simulink model "sistim"  (R2016a)
settings: Solver=FixedStepAuto  StartTime=0.0  StopTime=10.0  RelTol=1e-3
undefined symbols (not defined in the file): intellegent_control, LED_control, sigbuilder_block
libraries: fuzblock x2
settings Model: Creator=USER  LastModifiedBy=USER

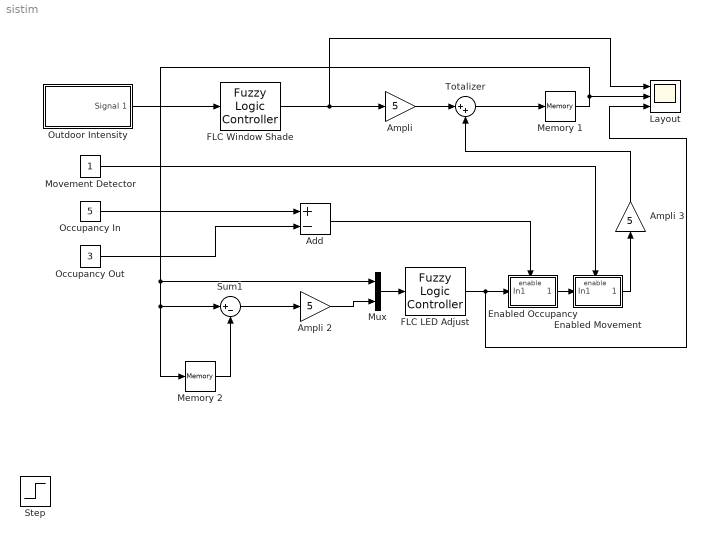
== system sistim ==
  "                     Totalizer" : Sum  Inputs=|++
  Add : Sum  Inputs=+-
  Ampli : Gain  Gain=5
  Ampli 2 : Gain  Gain=5
  Ampli 3 : Gain  Gain=5
  Enabled Movement : Subsystem  TreatAsAtomicUnit=on
  Enabled Occupancy : Subsystem  TreatAsAtomicUnit=on
  FLC LED Adjust : fuzblock/Fuzzy Logic  Controller  fis=[LED_control]
  FLC Window Shade : fuzblock/Fuzzy Logic  Controller  fis=[intellegent_control]
  Layout : Scope  NumInputPorts=3
  Memory 1 : Memory
  Memory 2 : Memory
  "Movement Detector " : Constant
  Mux : Mux  Inputs=2
  "Occupancy In " : Constant  Value=5
  Occupancy Out : Constant  Value=3
  Outdoor Intensity : Subsystem  Tag=STV Subsys  LoadFcn=sigbuilder_block('load');  StartFcn=sigbuilder_block('start');  StopFcn=sigbuilder_block('stop');  ClipboardFcn=sigbuilder_block('clipboard');  mask(Sigbuilder block){}
      mask help: Simulink:masks:SigbuilderBlock_MD
      mask init:
      | if ~strcmp(get_param(bdroot(gcbh),'SimulationStatus'),'stopped') tuvar = sigbuilder_block('maskInit'); end
      settings: CopyFcn=sigbuilder_block('copy');  DeleteFcn=sigbuilder_block('delete');  ModelCloseFcn=sigbuilder_block('modelClose');  PreSaveFcn=sigbuilder_block('preSave');  PauseFcn=sigbuilder_block('pause');  ContinueFcn=sigbuilder_block('continue');  NameChangeFcn=sigbuilder_block('namechange');  OpenFcn=sigbuilder_block('open',[317.25 117 550.5 359.25 ]);  CloseFcn=sigbuilder_block('close');
      mask Display: plot(0, 0, 100, 100,[2, 2, 32, 32, 2], [68, 8, 8, 68, 68],[32, 2], [38, 38], [32, 19, 2],[53, 60, 44], [32, 17, 17, 2],[16, 16, 31, 31]);txt = getActiveGroup(gcbh);text(2, 100, txt,'verticalAlignment', 'top');
  Step : Step  SampleTime=0
  Sum1 : Sum  Inputs=|+-
  wires:
  FLC Window Shade/1 -> Layout/1, Ampli/1
  "                     Totalizer"/1 -> Memory 1/1
  "Occupancy In "/1 -> Add/1
  Occupancy Out/1 -> Add/2
  Enabled Occupancy/1(Out1) -> Enabled Movement/1(In1)
  Add/1 -> Enabled Occupancy/Enable
  "Movement Detector "/1 -> Enabled Movement/Enable
  Mux/1 -> FLC LED Adjust/1
  Memory 2/1 -> Sum1/2
  Memory 1/1 -> Layout/2, Memory 2/1, Sum1/1, Mux/1
  Ampli 2/1 -> Mux/2
  Sum1/1 -> Ampli 2/1
  Enabled Movement/1(Out1) -> Ampli 3/1
  Ampli 3/1 -> "                     Totalizer"/2
  Ampli/1 -> "                     Totalizer"/1
  FLC LED Adjust/1 -> Layout/3, Enabled Occupancy/1(In1)
  Outdoor Intensity/1(Signal 1) -> FLC Window Shade/1

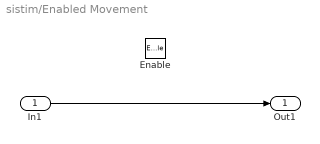
== system sistim/Enabled Movement ==
  In1 : Inport
  Enable : EnablePort
  Out1 : Outport
  wires:
  In1/1 -> Out1/1

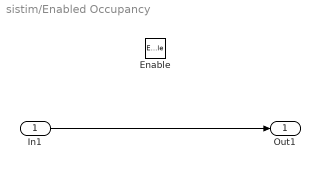
== system sistim/Enabled Occupancy ==
  In1 : Inport
  Enable : EnablePort
  Out1 : Outport
  wires:
  In1/1 -> Out1/1

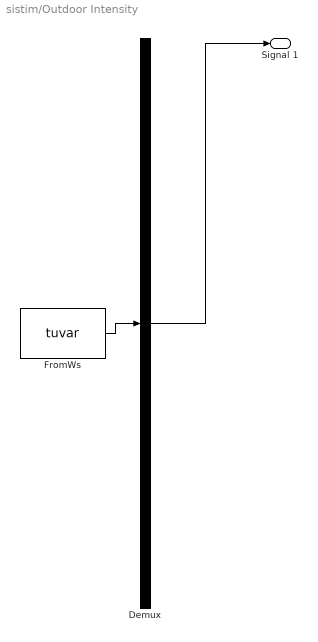
== system sistim/Outdoor Intensity ==
  Demux : Demux  Tag=STV Demux  Outputs=1
  FromWs : FromWorkspace  Tag=STV FromWs  VariableName=tuvar  SampleTime=0
      SigBuilderData=|
      | common.afterFinalStr = 'Extrapolate'
      | common.sampleTime = 0
      | dataSet.timeRange = [0 10]
      | dataSet.name = 'Group 1'
      | sbobj.Groups.Name = 'Group 1'
      | sbobj.Groups.Signals.Name = 'Signal 1'
      | sbobj.Groups.Signals.XData = [0 0.125 0.25 0.375 0.5 0.625 0.75 0.875 1 1.125 1.25 1.375 1.5 1.625 1.75 1.875 2 2.125 2.25 2.375 2.5 2.625 2.75 2.875 3 3.125 3.25 3.375 3.5 3.625 3.75 3.875 4 4.125 4.25 4.375 4.5 4.625 4.75 4.875 5 5.125 5.25 5.375 5.5 5.625 5.75 5.875 6 6.125 6.25 6.375 6.5 6.625 6.75 6.875 7 7.125 7.25 7.375 7.5 7.625 7.75 7.875 8 8.125 8.25 8.375 8.5 8.625 8.75 8.875 9 9.125 9.25 9.375 9.5 9.625 9.75 9.875 10]
      | sbobj.Groups.Signals.YData = [1 1.70710678119 2 1.70710678119 1 0.292893218813 0 0.292893218813 1 1.70710678119 2 1.70710678119 1 0.292893218813 0 0.292893218813 1 1.70710678119 2 1.70710678119 1 0.292893218813 0 0.292893218813 1 1.70710678119 2 1.70710678119 1 0.292893218813 0 0.292893218813 1 1.70710678119 2 1.70710678119 1 0.292893218813 0 0.292893218813 1 1.70710678119 2 1.70710678119 1 0.292893218813 0 0.292893218813 1 1.70710678119 2 1.70710678119 1 0.292893218813 0 0.292893218813 1 1.70710678119 2 1.70710678119 1 0.292893218813 0 0.292893218813 1 1.70710678119 2 1.70710678119 1 0.292893218813 0 0.292893218813 1 1.70710678119 2 1.70710678119 1 0.292893218813 0 0.292893218813 1]
  Signal 1 : Outport  Tag=STV Outport
  wires:
  Demux/1 -> Signal 1/1
  FromWs/1 -> Demux/1
